simulink model "sim2"  (R2021b)
settings: Solver=VariableStepAuto  StartTime=0.0  StopTime=50  RelTol=1e-3
settings Model: Creator=dcheb  LastModifiedBy=dcheb

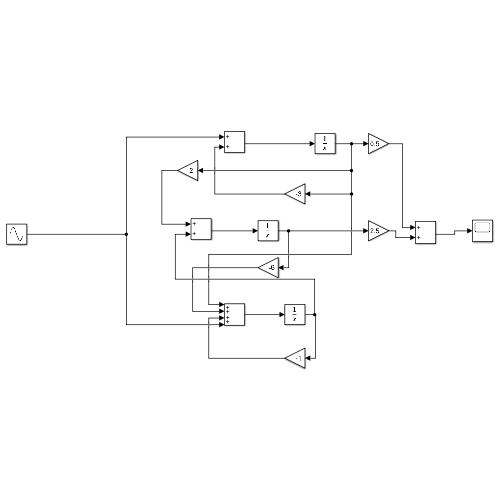
[thumbnail: Simulink's stored preview of the top-level diagram]
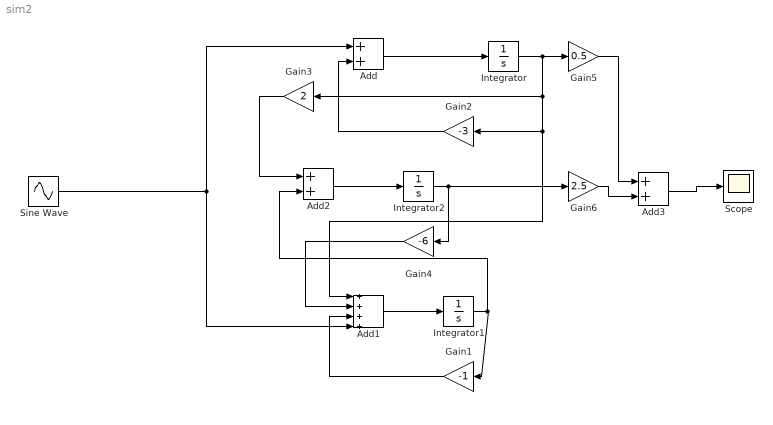
== system sim2 ==
  Add : Sum
  Add1 : Sum  Inputs=++++
  Add2 : Sum
  Add3 : Sum
  Gain1 : Gain  Gain=-1
  Gain2 : Gain  Gain=-3
  Gain3 : Gain  Gain=2
  Gain4 : Gain  Gain=-6
  Gain5 : Gain  Gain=0.5
  Gain6 : Gain  Gain=2.5
  Integrator : Integrator
  Integrator1 : Integrator
  Integrator2 : Integrator
  Scope : Scope
  Sine Wave : Sin  Amplitude=2  SampleTime=0
  wires:
  Sine Wave/1 -> Add1/4, Add/1
  Add/1 -> Integrator/1
  Integrator/1 -> Add1/1, Gain2/1, Gain3/1, Gain5/1
  Gain2/1 -> Add/2
  Add1/1 -> Integrator1/1
  Integrator1/1 -> Gain1/1, Add2/2
  Gain1/1 -> Add1/3
  Gain3/1 -> Add2/1
  Add2/1 -> Integrator2/1
  Integrator2/1 -> Gain4/1, Gain6/1
  Gain4/1 -> Add1/2
  Add3/1 -> Scope/1
  Gain5/1 -> Add3/1
  Gain6/1 -> Add3/2
